simulink model "Motor_ctrl_INST"  (R2025b)
settings: Solver=ode15s  StartTime=0.0  StopTime=1  FixedStep=Ts/10  MaxStep=Tstep  RelTol=1e-3  AbsTol=1e-3  EnableMultiTasking=on
InitFcn:
  | if ~exist('flagwp')
  |     tic
  |     init_sim
  | end
  | mex Motor_ctrl.c User_functions/Src/*.c
StopFcn:
  | if ~exist('flagwp')
  |   elapsed_time=toc
  | end
values from neighbouring files (symbols this model uses):
  accel = 5000    [init_sim.m]
  Bm = 0    [init_sim.m]
  Clarke_inv = [1 0;-0.5 sqrt(3)/2;-0.5 -sqrt(3)/2]    [init_sim.m]
  Ctrl_strategy = 1    [init_sim.m]
  Ctrl_type = 3    [init_sim.m]
  dem = 1    [init_sim.m]
  dT = motorModel.SyreDrive.Converter.dT * 1e-6    [init_sim.m]
  expC = motorModel.IronPMLossMap_dq.expC    [init_sim.m]
  expH = motorModel.IronPMLossMap_dq.expH    [init_sim.m]
  expPM = motorModel.IronPMLossMap_dq.expPM    [init_sim.m]
  Fd0 = interp2(motorModel.FluxMap_dq.Id,motorModel.FluxMap_dq.Iq,motorModel.FluxMap_dq.Fd,0,0)    [init_sim.m]
  Fm = interp2(Idd,Iqq,Fdd,0,0)    [init_sim.m]
  HS_ctrl = 1    [init_sim.m]
  Id_dqt = interpn(motorModel.FluxMapInv_dqt.dataF.Fd,motorModel.FluxMapInv_dqt.dataF.Fq,motorModel.FluxMapInv_dqt.dataF.th,motorModel.FluxMapInv_dqt.dataF.Id,Fd_dqt,Fq_dqt,th_dqt,'cubic')    [init_sim.m]
  Id_fe = motorModel.IronPMLossMap_dq.Id    [init_sim.m]
  InitIntg_d = Fm*cos(th0)    [init_sim.m]
  InitIntg_q = Fm*sin(th0)    [init_sim.m]
  inj_waveform = 1    [init_sim.m]
  Iq_dqt = interpn(motorModel.FluxMapInv_dqt.dataF.Fd,motorModel.FluxMapInv_dqt.dataF.Fq,motorModel.FluxMapInv_dqt.dataF.th,motorModel.FluxMapInv_dqt.dataF.Iq,Fd_dqt,Fq_dqt,th_dqt,'cubic')    [init_sim.m]
  Iq_fe = motorModel.IronPMLossMap_dq.Iq    [init_sim.m]
  IronLoss = 1    [init_sim.m]
  J = motorModel.data.J    [init_sim.m]
  n0 = motorModel.IronPMLossMap_dq.n0    [init_sim.m]
  p = motorModel.data.p    [init_sim.m]
  Pfe_c = motorModel.IronPMLossMap_dq.Pfes_c + motorModel.IronPMLossMap_dq.Pfer_c    [init_sim.m]
  Pfe_h = motorModel.IronPMLossMap_dq.Pfes_h + motorModel.IronPMLossMap_dq.Pfer_h    [init_sim.m]
  Ppm = motorModel.IronPMLossMap_dq.Ppm    [init_sim.m]
  Quad_Maps = 2    [init_sim.m]
  SS_on = 1    [init_sim.m]
  T_dqt = interpn(motorModel.FluxMapInv_dqt.dataF.Fd,motorModel.FluxMapInv_dqt.dataF.Fq,motorModel.FluxMapInv_dqt.dataF.th,motorModel.FluxMapInv_dqt.dataF.T,Fd_dqt,Fq_dqt,th_dqt,'cubic')    [init_sim.m]
  Tf = 0    [init_sim.m]
  th0 = 0    [init_sim.m]
  th_max = max(motorModel.FluxMapInv_dqt.dataF.th,[],'all')    [init_sim.m]
  th_min = min(motorModel.FluxMapInv_dqt.dataF.th,[],'all')    [init_sim.m]
  Ts = 1/motorModel.SyreDrive.Converter.fPWM    [init_sim.m]
  Tv = 0    [init_sim.m]
  VDC = motorModel.data.Vdc    [init_sim.m]
undefined symbols (not defined in the file or in its folder): ACloss, eMotor, fD_pu_norm, fD_vct_max, fD_vct_ref, fQ_pu_norm, fQ_vct_max, fQ_vct_ref, iD_pu_norm, idRef, interpn, iQ_pu_norm, iqRef, J_rot, magnitude, motorModelType, nRef, sigbuilder_block, T0
libraries: nesl_utility x43, fl_lib x41, ee_lib x8, simulink x8, eeTransforms x1
(part 3 of 4)

== system Motor_ctrl_INST/Power block - Inverter + Motor/Circuital/Motor model/CCG model/Motor Model/Rs2/no AC loss ==
  Rs : Inport
  Current Sensor : fl_lib/Electrical/Electrical Sensors/Current Sensor
  PS-Simulink Converter : nesl_utility/PS-Simulink Converter  PhysicalDomain=network_engine_domain  SubClassName=ps_output  LeftPortType=input  RightPortType=output  PseudoPeriodic=off  Frequencies=[]  VectorFormat=inherit  Unit=inherit  AffineConversion=off
  PS-Simulink Converter1 : nesl_utility/PS-Simulink Converter  PhysicalDomain=network_engine_domain  SubClassName=ps_output  LeftPortType=input  RightPortType=output  PseudoPeriodic=off  Frequencies=[]  VectorFormat=inherit  Unit=inherit  AffineConversion=off
  Product : Product
  Resistor : fl_lib/Electrical/Electrical Elements/Resistor  R=ACloss.Rac(1) Ohm  i_specify=off  i_priority=None  i=0 A  i_nominal_specify=off  i_nominal_value=1  i_nominal_unit=A  v_specify=off  v_priority=None  v=0 V  v_nominal_specify=off  v_nominal_value=1  v_nominal_unit=V
  Terminator : Terminator
  Voltage Sensor : fl_lib/Electrical/Electrical Sensors/Voltage Sensor
  In : PMIOPort  Side=Left
  Out : PMIOPort  Port=2  Side=Right
  Pjs : Outport
  wires:
  PS-Simulink Converter/1 -> Product/1
  PS-Simulink Converter1/1 -> Product/2
  Product/1 -> Pjs/1
  Rs/1 -> Terminator/1
  connections:
  Resistor/LConn1 -- In/RConn1 -- Voltage Sensor/LConn1
  Current Sensor/RConn2 -- Out/RConn1
  Resistor/RConn1 -- Current Sensor/LConn1 -- Voltage Sensor/RConn2
  PS-Simulink Converter/LConn1 -- Voltage Sensor/RConn1
  PS-Simulink Converter1/LConn1 -- Current Sensor/RConn1

== system Motor_ctrl_INST/Power block - Inverter + Motor/Circuital/Motor model/CCG model/Motor Model/Rs2/yes AC loss ==
  Rs : Inport
  Current Sensor : fl_lib/Electrical/Electrical Sensors/Current Sensor
  PS-Simulink Converter : nesl_utility/PS-Simulink Converter  PhysicalDomain=network_engine_domain  SubClassName=ps_output  LeftPortType=input  RightPortType=output  PseudoPeriodic=off  Frequencies=[]  VectorFormat=inherit  Unit=inherit  AffineConversion=off
  PS-Simulink Converter1 : nesl_utility/PS-Simulink Converter  PhysicalDomain=network_engine_domain  SubClassName=ps_output  LeftPortType=input  RightPortType=output  PseudoPeriodic=off  Frequencies=[]  VectorFormat=inherit  Unit=inherit  AffineConversion=off
  Product : Product
  Simulink-PS Converter : nesl_utility/Simulink-PS Converter  PhysicalDomain=network_engine_domain  SubClassName=ps_input  LeftPortType=input  RightPortType=output  PseudoPeriodic=off  Frequencies=[]  NoiseDistribution=none  NoiseParameters=[]  Unit=1  AffineConversion=off  FilteringAndDerivatives=provide  SimscapeFilterOrder=1  InputFilterTimeConstant=0.001  UdotUserProvided=0
  Variable Resistor : fl_lib/Electrical/Electrical Elements/Variable Resistor  Rmin=0 Ohm  thermalEnable=false  thermal_mass=1 J/K  i_specify=off  i_priority=None  i=0 A  i_nominal_specify=off  i_nominal_value=1  i_nominal_unit=A  v_specify=off  v_priority=None  v=0 V  v_nominal_specify=off  v_nominal_value=1  v_nominal_unit=V  T_specify=off  T_priority=None  T=300 K  T_nominal_specify=off  T_nominal_value=1  T_nominal_unit=K
  Voltage Sensor : fl_lib/Electrical/Electrical Sensors/Voltage Sensor
  In : PMIOPort  Side=Left
  Out : PMIOPort  Port=2  Side=Right
  Pjs : Outport
  wires:
  PS-Simulink Converter1/1 -> Product/2
  PS-Simulink Converter/1 -> Product/1
  Product/1 -> Pjs/1
  Rs/1 -> Simulink-PS Converter/1
  connections:
  Variable Resistor/RConn1 -- Current Sensor/LConn1 -- Voltage Sensor/RConn2
  In/RConn1 -- Voltage Sensor/LConn1 -- Variable Resistor/LConn2
  Current Sensor/RConn2 -- Out/RConn1
  PS-Simulink Converter1/LConn1 -- Current Sensor/RConn1
  PS-Simulink Converter/LConn1 -- Voltage Sensor/RConn1
  Variable Resistor/LConn1 -- Simulink-PS Converter/RConn1

== system Motor_ctrl_INST/Power block - Inverter + Motor/Noncircuital/FM/Motor Model/Inverse Flux Maps/2D LUT/dq Model ==
  note: 1) Add Subsystem or Model blocks as valid variant choices.
      | 2) You cannot connect blocks at this level. At simulation, connectivity is automatically
      | determined, based on the active variant and port name matching.
  Vabc : Inport
  theta_elt : Inport  Port=2
  we : Inport  Port=3
  IPM : Subsystem  VariantControl=Quad_Maps==2
  PM-SyR : Subsystem  VariantControl=Quad_Maps==1
  SyR : Subsystem  VariantControl=Quad_Maps==0
  idq : Outport
  T : Outport  Port=2
  i0 : Outport  Port=3
  Fdq : Outport  Port=4

== system Motor_ctrl_INST/Power block - Inverter + Motor/Noncircuital/FM/Motor Model/Inverse Flux Maps/3D LUTs/Variant Subsystem ==
  note: 1) Add Subsystem or Model blocks as valid variant choices.
      | 2) You cannot connect blocks at this level. At simulation, connectivity is automatically
      | determined, based on the active variant and port name matching.
  Vabc : Inport
  theta_elt : Inport  Port=2
  we : Inport  Port=3
  IPM : Subsystem  VariantControl=Quad_Maps==2
  PM-SyR : Subsystem  VariantControl=Quad_Maps==1
  SyR : Subsystem  VariantControl=Quad_Maps==0
  idq : Outport
  T : Outport  Port=2
  i0 : Outport  Port=3
  Fdq : Outport  Port=4

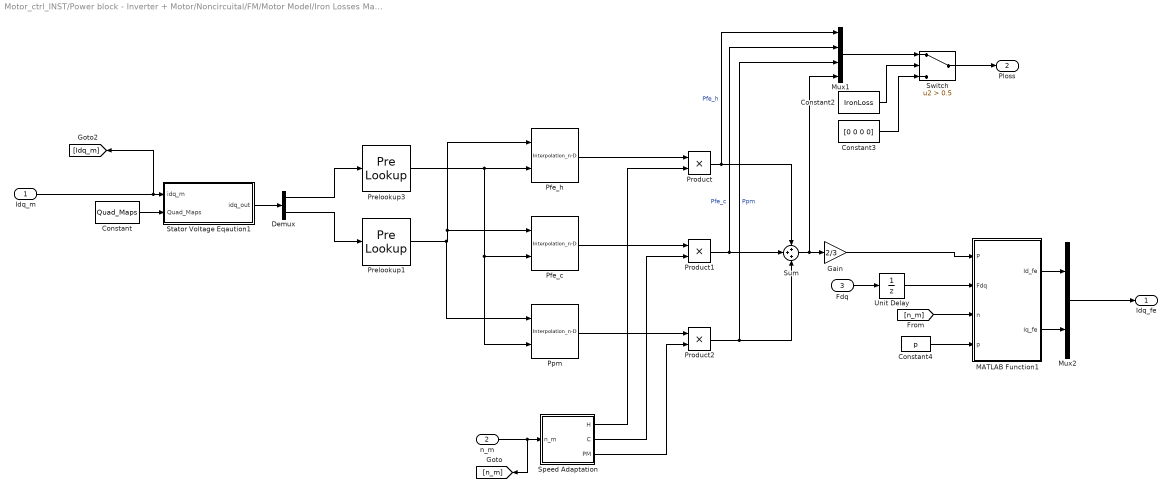
== system Motor_ctrl_INST/Power block - Inverter + Motor/Noncircuital/FM/Motor Model/Iron Losses Maps/Iron Losses/Iron loss Maps ==
  Idq_m : Inport
  n_m : Inport  Port=2
  Fdq : Inport  Port=3
  Constant : Constant  Value=Quad_Maps
  Constant2 : Constant  Value=IronLoss
  Constant3 : Constant  Value=[0 0 0 0]
  Constant4 : Constant  Value=p
  Demux : Demux  Outputs=2
  Gain : Gain  Gain=2/3
  MATLAB Function1 : MATLAB Function  TreatAsAtomicUnit=on
  Mux1 : Mux
  Mux2 : Mux  Inputs=2
  Pfe_c : Interpolation_n-D  Table=Pfe_c  RequireIndexFractionAsBus=on  InternalRulePriority=Speed
      settings: InputPortMap=u0,u1
  Pfe_h : Interpolation_n-D  Table=Pfe_h  RequireIndexFractionAsBus=on  InternalRulePriority=Speed
      settings: InputPortMap=u0,u1
  Ppm : Interpolation_n-D  Table=Ppm  RequireIndexFractionAsBus=on  InternalRulePriority=Speed
      settings: InputPortMap=u0,u1
  Prelookup1 : PreLookup  BreakpointsData=Iq_fe(:,1)  OutputSelection=Index and fraction as bus  ExtrapMethod=Linear
  Prelookup3 : PreLookup  BreakpointsData=Id_fe(1,:)  OutputSelection=Index and fraction as bus  ExtrapMethod=Linear
  Product : Product
  Product1 : Product
  Product2 : Product
  Speed Adaptation : Subsystem
  Stator Voltage Eqaution1 : MATLAB Function  TreatAsAtomicUnit=on
  Sum : Sum  Inputs=+++
  Switch : Switch  Criteria=u2 > Threshold  Threshold=0.5  SaturateOnIntegerOverflow=off  InputSameDT=off
  Unit Delay : UnitDelay  SampleTime=-1  HasFrameUpgradeWarning=on
  Idq_fe : Outport
  Ploss : Outport  Port=2
  wires:
  Product1/1 -> Mux1/2, Sum/2  "Pfe_c"
  Product2/1 -> Mux1/3, Sum/3  "Ppm"
  Pfe_h/1 -> Product/1
  Prelookup3/1 -> Ppm/2, Pfe_c/2, Pfe_h/2
  Speed Adaptation/1(H) -> Product/2
  n_m/1 -> Speed Adaptation/1(n_m), [n_m]
  Demux/1 -> Prelookup3/1
  Sum/1 -> Mux1/4, Gain/1
  Product/1 -> Sum/1, Mux1/1  "Pfe_h"
  Speed Adaptation/2(C) -> Product1/2
  Prelookup1/1 -> Ppm/1, Pfe_h/1, Pfe_c/1
  Pfe_c/1 -> Product1/1
  Ppm/1 -> Product2/1
  Demux/2 -> Prelookup1/1
  Speed Adaptation/3(PM) -> Product2/2
  Constant/1 -> Stator Voltage Eqaution1/2(Quad_Maps)
  Stator Voltage Eqaution1/1(idq_out) -> Demux/1
  Idq_m/1 -> [Idq_m], Stator Voltage Eqaution1/1(idq_m)
  Gain/1 -> MATLAB Function1/1(P)
  Fdq/1 -> Unit Delay/1
  [n_m] -> MATLAB Function1/3(n)
  Constant4/1 -> MATLAB Function1/4(p)
  MATLAB Function1/1(Id_fe) -> Mux2/1
  Mux2/1 -> Idq_fe/1
  Unit Delay/1 -> MATLAB Function1/2(Fdq)
  MATLAB Function1/2(Iq_fe) -> Mux2/2
  Mux1/1 -> Switch/1
  Constant2/1 -> Switch/2
  Switch/1 -> Ploss/1
  Constant3/1 -> Switch/3

== system Motor_ctrl_INST/Power block - Inverter + Motor/Circuital/Motor model/CCG model/Motor Model/Inverse Flux Maps/2D LUT/dq Model ==
  note: 1) Add Subsystem or Model blocks as valid variant choices.
      | 2) You cannot connect blocks at this level. At simulation, connectivity is automatically
      | determined, based on the active variant and port name matching.
  Fdq : Inport
  IPM : Subsystem  VariantControl=Quad_Maps==2
  PM-SyR : Subsystem  VariantControl=Quad_Maps==1
  SyR : Subsystem  VariantControl=Quad_Maps==0
  idq : Outport
  T : Outport  Port=2

== system Motor_ctrl_INST/Power block - Inverter + Motor/Circuital/Motor model/CCG model/Motor Model/Inverse Flux Maps/3D LUTs/Variant Subsystem ==
  note: 1) Add Subsystem or Model blocks as valid variant choices.
      | 2) You cannot connect blocks at this level. At simulation, connectivity is automatically
      | determined, based on the active variant and port name matching.
  Fdq : Inport
  theta_elt : Inport  Port=2
  IPM : Subsystem  VariantControl=Quad_Maps==2
  PM-SyR : Subsystem  VariantControl=Quad_Maps==1
  SyR : Subsystem  VariantControl=Quad_Maps==0
  idq : Outport
  T : Outport  Port=2

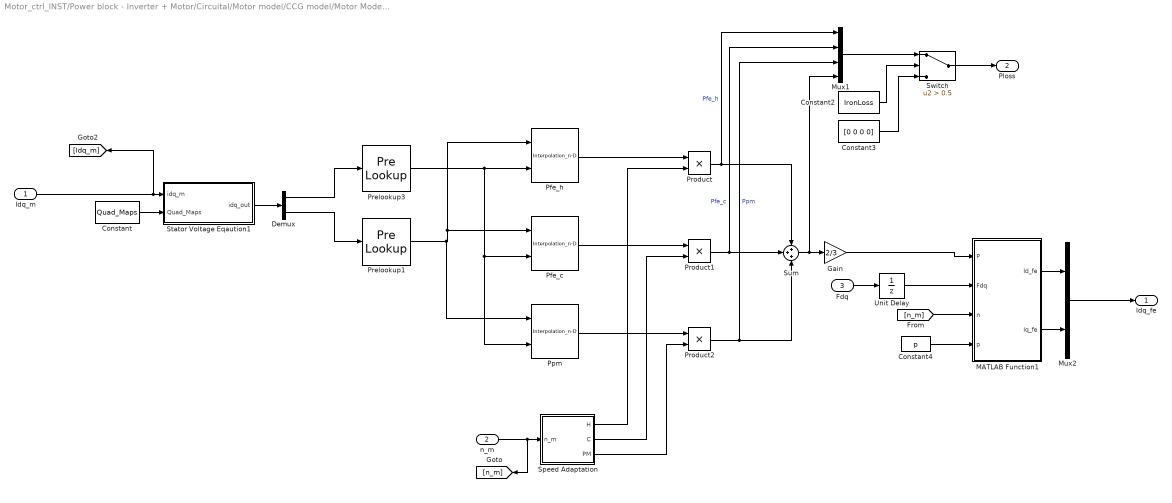
== system Motor_ctrl_INST/Power block - Inverter + Motor/Circuital/Motor model/CCG model/Motor Model/Iron Losses Maps/Iron Losses/Iron loss Maps ==
  Idq_m : Inport
  n_m : Inport  Port=2
  Fdq : Inport  Port=3
  Constant : Constant  Value=Quad_Maps
  Constant2 : Constant  Value=IronLoss
  Constant3 : Constant  Value=[0 0 0 0]
  Constant4 : Constant  Value=p
  Demux : Demux  Outputs=2
  Gain : Gain  Gain=2/3
  MATLAB Function1 : MATLAB Function  TreatAsAtomicUnit=on
  Mux1 : Mux
  Mux2 : Mux  Inputs=2
  Pfe_c : Interpolation_n-D  Table=Pfe_c  RequireIndexFractionAsBus=on  InternalRulePriority=Speed
      settings: InputPortMap=u0,u1
  Pfe_h : Interpolation_n-D  Table=Pfe_h  RequireIndexFractionAsBus=on  InternalRulePriority=Speed
      settings: InputPortMap=u0,u1
  Ppm : Interpolation_n-D  Table=Ppm  RequireIndexFractionAsBus=on  InternalRulePriority=Speed
      settings: InputPortMap=u0,u1
  Prelookup1 : PreLookup  BreakpointsData=Iq_fe(:,1)  OutputSelection=Index and fraction as bus  ExtrapMethod=Linear
  Prelookup3 : PreLookup  BreakpointsData=Id_fe(1,:)  OutputSelection=Index and fraction as bus  ExtrapMethod=Linear
  Product : Product
  Product1 : Product
  Product2 : Product
  Speed Adaptation : Subsystem
  Stator Voltage Eqaution1 : MATLAB Function  TreatAsAtomicUnit=on
  Sum : Sum  Inputs=+++
  Switch : Switch  Criteria=u2 > Threshold  Threshold=0.5  SaturateOnIntegerOverflow=off  InputSameDT=off
  Unit Delay : UnitDelay  SampleTime=-1  HasFrameUpgradeWarning=on
  Idq_fe : Outport
  Ploss : Outport  Port=2
  wires:
  Product1/1 -> Mux1/2, Sum/2  "Pfe_c"
  Product2/1 -> Mux1/3, Sum/3  "Ppm"
  Pfe_h/1 -> Product/1
  Prelookup3/1 -> Ppm/2, Pfe_c/2, Pfe_h/2
  Speed Adaptation/1(H) -> Product/2
  n_m/1 -> Speed Adaptation/1(n_m), [n_m]
  Demux/1 -> Prelookup3/1
  Sum/1 -> Mux1/4, Gain/1
  Product/1 -> Sum/1, Mux1/1  "Pfe_h"
  Speed Adaptation/2(C) -> Product1/2
  Prelookup1/1 -> Ppm/1, Pfe_h/1, Pfe_c/1
  Pfe_c/1 -> Product1/1
  Ppm/1 -> Product2/1
  Demux/2 -> Prelookup1/1
  Speed Adaptation/3(PM) -> Product2/2
  Constant/1 -> Stator Voltage Eqaution1/2(Quad_Maps)
  Stator Voltage Eqaution1/1(idq_out) -> Demux/1
  Idq_m/1 -> [Idq_m], Stator Voltage Eqaution1/1(idq_m)
  Gain/1 -> MATLAB Function1/1(P)
  Fdq/1 -> Unit Delay/1
  [n_m] -> MATLAB Function1/3(n)
  Constant4/1 -> MATLAB Function1/4(p)
  MATLAB Function1/1(Id_fe) -> Mux2/1
  Mux2/1 -> Idq_fe/1
  Unit Delay/1 -> MATLAB Function1/2(Fdq)
  MATLAB Function1/2(Iq_fe) -> Mux2/2
  Mux1/1 -> Switch/1
  Constant2/1 -> Switch/2
  Switch/1 -> Ploss/1
  Constant3/1 -> Switch/3

== system Motor_ctrl_INST/Power block - Inverter + Motor/Noncircuital/FM/Motor Model/Inverse Flux Maps/2D LUT/dq Model/IPM ==
  Vabc : Inport
  theta_elt : Inport  Port=2
  we : Inport  Port=3
  Add : Sum  Inputs=-+-
  Constant : Constant  Value=0
  Demux1 : Demux  Outputs=3
  "Fdq -> idq" : Subsystem
  Gain1 : Gain  Gain=J_rot  Multiplication=Matrix(K*u)
  Gain3 : Gain  Gain=1/p
  Integrator : Integrator  InitialCondition=[Fd0 0]
  Mux1 : Mux  Inputs=2
  Product : Product
  Product2 : Product
  Subsystem1 : Subsystem
  Terminator : Terminator
  ab->dq1 : Subsystem
      mask Display: disp('A(-theta)')
  abc->ab0 : Subsystem
  idq : Outport
  T : Outport  Port=2
  i0 : Outport  Port=3
  Fdq : Outport  Port=4
  wires:
  Add/1 -> Integrator/1
  Demux1/2 -> Mux1/2
  we/1 -> Product/2
  [Rs] -> Product2/1
  Product2/1 -> Add/1
  "Fdq -> idq"/2(T) -> T/1
  Demux1/1 -> Mux1/1
  abc->ab0/1(eab0) -> Demux1/1
  "Fdq -> idq"/1(idq) -> Product2/2, idq/1
  Product/1 -> Add/3
  theta_elt/1 -> Gain3/1
  ab->dq1/1(X_dq) -> Add/2
  Vabc/1 -> abc->ab0/1(eabc)
  Integrator/1 -> "Fdq -> idq"/1(Fdq), Fdq/1, Gain1/1
  Gain3/1 -> Subsystem1/1(theta_r)
  Mux1/1 -> ab->dq1/1(X_ab)
  Gain1/1 -> Product/1
  Subsystem1/1(SinCos) -> ab->dq1/2(sin,cos)
  Constant/1 -> i0/1
  Demux1/3 -> Terminator/1

== system Motor_ctrl_INST/Power block - Inverter + Motor/Noncircuital/FM/Motor Model/Inverse Flux Maps/2D LUT/dq Model/PM-SyR ==
  Vabc : Inport
  theta_elt : Inport  Port=2
  we : Inport  Port=3
  Add : Sum  Inputs=-+-
  Constant : Constant  Value=0
  Demux1 : Demux  Outputs=3
  "Fdq -> idq" : Subsystem
  Gain1 : Gain  Gain=J_rot  Multiplication=Matrix(K*u)
  Gain3 : Gain  Gain=1/p
  Integrator : Integrator  InitialCondition=[Fd0 0]
  Mux1 : Mux  Inputs=2
  Product : Product
  Product2 : Product
  Subsystem1 : Subsystem
  Terminator : Terminator
  ab->dq1 : Subsystem
      mask Display: disp('A(-theta)')
  abc->ab0 : Subsystem
  idq : Outport
  T : Outport  Port=2
  i0 : Outport  Port=3
  Fdq : Outport  Port=4
  wires:
  Subsystem1/1(SinCos) -> ab->dq1/2(sin,cos)
  Product/1 -> Add/3
  theta_elt/1 -> Gain3/1
  Mux1/1 -> ab->dq1/1(X_ab)
  Integrator/1 -> "Fdq -> idq"/1(Fdq), Fdq/1, Gain1/1
  Gain1/1 -> Product/1
  Vabc/1 -> abc->ab0/1(eabc)
  Gain3/1 -> Subsystem1/1(theta_r)
  ab->dq1/1(X_dq) -> Add/2
  abc->ab0/1(eab0) -> Demux1/1
  "Fdq -> idq"/1(idq) -> Product2/2, idq/1
  Demux1/1 -> Mux1/1
  Add/1 -> Integrator/1
  [Rs] -> Product2/1
  Demux1/2 -> Mux1/2
  Product2/1 -> Add/1
  we/1 -> Product/2
  "Fdq -> idq"/2(T) -> T/1
  Constant/1 -> i0/1
  Demux1/3 -> Terminator/1

== system Motor_ctrl_INST/Power block - Inverter + Motor/Noncircuital/FM/Motor Model/Inverse Flux Maps/2D LUT/dq Model/SyR ==
  Vabc : Inport
  theta_elt : Inport  Port=2
  we : Inport  Port=3
  Add : Sum  Inputs=-+-
  Constant : Constant  Value=0
  Demux1 : Demux  Outputs=3
  "Fdq -> idq" : Subsystem
  Gain1 : Gain  Gain=J_rot  Multiplication=Matrix(K*u)
  Gain3 : Gain  Gain=1/p
  Integrator : Integrator  InitialCondition=[Fd0 0]
  Mux1 : Mux  Inputs=2
  Product : Product
  Product2 : Product
  Subsystem1 : Subsystem
  Terminator : Terminator
  ab->dq1 : Subsystem
      mask Display: disp('A(-theta)')
  abc->ab0 : Subsystem
  idq : Outport
  T : Outport  Port=2
  i0 : Outport  Port=3
  Fdq : Outport  Port=4
  wires:
  Subsystem1/1(SinCos) -> ab->dq1/2(sin,cos)
  Product/1 -> Add/3
  theta_elt/1 -> Gain3/1
  Mux1/1 -> ab->dq1/1(X_ab)
  Integrator/1 -> "Fdq -> idq"/1(Fdq), Fdq/1, Gain1/1
  Gain1/1 -> Product/1
  Vabc/1 -> abc->ab0/1(eabc)
  Gain3/1 -> Subsystem1/1(theta_r)
  ab->dq1/1(X_dq) -> Add/2
  abc->ab0/1(eab0) -> Demux1/1
  "Fdq -> idq"/1(idq) -> Product2/2, idq/1
  Demux1/1 -> Mux1/1
  Add/1 -> Integrator/1
  [Rs] -> Product2/1
  Demux1/2 -> Mux1/2
  "Fdq -> idq"/2(T) -> T/1
  Product2/1 -> Add/1
  we/1 -> Product/2
  Constant/1 -> i0/1
  Demux1/3 -> Terminator/1

== system Motor_ctrl_INST/Power block - Inverter + Motor/Noncircuital/FM/Motor Model/Inverse Flux Maps/3D LUTs/Variant Subsystem/IPM ==
  Vabc : Inport
  theta_elt : Inport  Port=2
  we : Inport  Port=3
  Add : Sum  Inputs=-+-
  Constant : Constant  Value=0
  Demux1 : Demux  Outputs=3
  "Fdq -> idq" : Subsystem
      settings: PortSchema="{\"entries\":[{\"content\":{\"sides\":[{\"content\":{\"connectorIds\":[\"In1\"]},\"type\":\"ConnectorPlacement.EquallySpacedRectSide\",\"uuid\":\"c4c89702-6ed2-4f3f-ac47-63a7def21c28\"},{\"content\":{\"connectorIds\":[\"Out1\",\"Out2\"],\"side\":\"RIGHT\"},\"type\":\"ConnectorPlacement.EquallySpacedRectSide\",\"uuid\":\"78e6e96f-e01c-41b0-b9cc-2e557d2d3e77\"},{\"content\":{\"side\":\"TOP\"},\"type\":\"ConnectorPlacement.EquallySpacedRectSide\",\"uuid\":\"5ba1a012-9577-477d-841c-cd762f3f0080\"},{\"content\":{\"connectorIds\":[\"In2\"],\"side\":\"BOTTOM\"},\"type\":\"ConnectorPlacement.EquallySpacedRectSide\",\"uuid\":\"5a42fb6c-9e1a-4def-8312-83961c7d32ea\"}]},\"type\":\"ConnectorPlacement.EquallySpacedConnector\",\"uuid\":\"db03f8b0-b4f5-4aab-82fc-8dea803a4789\"}],\"packageUris\":[\"http://schema.mathworks.com/mf0/Connector/R2020b\"],\"version\":\"1.0\"}"
  Gain1 : Gain  Gain=J_rot  Multiplication=Matrix(K*u)
  Gain3 : Gain  Gain=1/p
  Integrator : Integrator  InitialCondition=[Fd0 0]
  Mux1 : Mux  Inputs=2
  Product : Product
  Product1 : Product
  Subsystem1 : Subsystem
  Terminator : Terminator
  ab->dq1 : Subsystem
      mask Display: disp('A(-theta)')
  abc->ab0 : Subsystem
  idq : Outport
  T : Outport  Port=2
  i0 : Outport  Port=3
  Fdq : Outport  Port=4
  wires:
  theta_elt/1 -> "Fdq -> idq"/2(th_e), Gain3/1
  Product1/1 -> Add/1
  Gain1/1 -> Product/1
  we/1 -> Product/2
  Product/1 -> Add/3
  Add/1 -> Integrator/1
  Integrator/1 -> Fdq/1, "Fdq -> idq"/1(Fdq), Gain1/1
  "Fdq -> idq"/1(idq) -> Product1/2, idq/1
  "Fdq -> idq"/2(T) -> T/1
  [Rs] -> Product1/1
  Vabc/1 -> abc->ab0/1(eabc)
  Gain3/1 -> Subsystem1/1(theta_r)
  abc->ab0/1(eab0) -> Demux1/1
  Subsystem1/1(SinCos) -> ab->dq1/2(sin,cos)
  Demux1/2 -> Mux1/2
  Mux1/1 -> ab->dq1/1(X_ab)
  Demux1/1 -> Mux1/1
  ab->dq1/1(X_dq) -> Add/2
  Constant/1 -> i0/1
  Demux1/3 -> Terminator/1

== system Motor_ctrl_INST/Power block - Inverter + Motor/Noncircuital/FM/Motor Model/Inverse Flux Maps/3D LUTs/Variant Subsystem/PM-SyR ==
  Vabc : Inport
  theta_elt : Inport  Port=2
  we : Inport  Port=3
  Add : Sum  Inputs=-+-
  Constant : Constant  Value=0
  Demux1 : Demux  Outputs=3
  "Fdq -> idq" : Subsystem
      settings: PortSchema="{\"entries\":[{\"content\":{\"sides\":[{\"content\":{\"connectorIds\":[\"In1\"]},\"type\":\"ConnectorPlacement.EquallySpacedRectSide\",\"uuid\":\"658e0025-c3b4-4188-99f2-cbeabc2b5232\"},{\"content\":{\"connectorIds\":[\"Out1\",\"Out2\"],\"side\":\"RIGHT\"},\"type\":\"ConnectorPlacement.EquallySpacedRectSide\",\"uuid\":\"553a685c-efe6-4f4b-af8f-d6d55fb3aed3\"},{\"content\":{\"side\":\"TOP\"},\"type\":\"ConnectorPlacement.EquallySpacedRectSide\",\"uuid\":\"e1cc6d12-3f22-4810-870a-14518fddf4c6\"},{\"content\":{\"connectorIds\":[\"In2\"],\"side\":\"BOTTOM\"},\"type\":\"ConnectorPlacement.EquallySpacedRectSide\",\"uuid\":\"8fa353db-c23e-4667-be44-c63eaefe25e8\"}]},\"type\":\"ConnectorPlacement.EquallySpacedConnector\",\"uuid\":\"5d87f386-f61d-410e-9580-edc792fe8ce3\"}],\"packageUris\":[\"http://schema.mathworks.com/mf0/Connector/R2020b\"],\"version\":\"1.0\"}"
  Gain1 : Gain  Gain=J_rot  Multiplication=Matrix(K*u)
  Gain3 : Gain  Gain=1/p
  Integrator : Integrator  InitialCondition=[Fd0 0]
  Mux1 : Mux  Inputs=2
  Product : Product
  Product1 : Product
  Subsystem1 : Subsystem
  Terminator : Terminator
  ab->dq1 : Subsystem
      mask Display: disp('A(-theta)')
  abc->ab0 : Subsystem
  idq : Outport
  T : Outport  Port=2
  i0 : Outport  Port=3
  Fdq : Outport  Port=4
  wires:
  we/1 -> Product/2
  Subsystem1/1(SinCos) -> ab->dq1/2(sin,cos)
  Mux1/1 -> ab->dq1/1(X_ab)
  Gain1/1 -> Product/1
  Product/1 -> Add/3
  abc->ab0/1(eab0) -> Demux1/1
  ab->dq1/1(X_dq) -> Add/2
  [Rs] -> Product1/1
  "Fdq -> idq"/2(T) -> T/1
  Demux1/1 -> Mux1/1
  Product1/1 -> Add/1
  Demux1/3 -> Terminator/1
  Gain3/1 -> Subsystem1/1(theta_r)
  Integrator/1 -> "Fdq -> idq"/1(Fdq), Fdq/1, Gain1/1
  "Fdq -> idq"/1(idq) -> Product1/2, idq/1
  Demux1/2 -> Mux1/2
  Add/1 -> Integrator/1
  Vabc/1 -> abc->ab0/1(eabc)
  theta_elt/1 -> Gain3/1, "Fdq -> idq"/2(theta_elt)
  Constant/1 -> i0/1

== system Motor_ctrl_INST/Power block - Inverter + Motor/Noncircuital/FM/Motor Model/Inverse Flux Maps/3D LUTs/Variant Subsystem/SyR ==
  Vabc : Inport
  theta_elt : Inport  Port=2
  we : Inport  Port=3
  Add : Sum  Inputs=-+-
  Constant : Constant  Value=0
  Demux1 : Demux  Outputs=3
  "Fdq -> idq" : Subsystem
      settings: PortSchema="{\"entries\":[{\"content\":{\"sides\":[{\"content\":{\"connectorIds\":[\"In1\"]},\"type\":\"ConnectorPlacement.EquallySpacedRectSide\",\"uuid\":\"658e0025-c3b4-4188-99f2-cbeabc2b5232\"},{\"content\":{\"connectorIds\":[\"Out1\",\"Out2\"],\"side\":\"RIGHT\"},\"type\":\"ConnectorPlacement.EquallySpacedRectSide\",\"uuid\":\"553a685c-efe6-4f4b-af8f-d6d55fb3aed3\"},{\"content\":{\"side\":\"TOP\"},\"type\":\"ConnectorPlacement.EquallySpacedRectSide\",\"uuid\":\"e1cc6d12-3f22-4810-870a-14518fddf4c6\"},{\"content\":{\"connectorIds\":[\"In2\"],\"side\":\"BOTTOM\"},\"type\":\"ConnectorPlacement.EquallySpacedRectSide\",\"uuid\":\"ed75ffcc-b3fe-4912-8b15-453be7565ae7\"}]},\"type\":\"ConnectorPlacement.EquallySpacedConnector\",\"uuid\":\"5d87f386-f61d-410e-9580-edc792fe8ce3\"}],\"packageUris\":[\"http://schema.mathworks.com/mf0/Connector/R2020b\"],\"version\":\"1.0\"}"
  Gain1 : Gain  Gain=J_rot  Multiplication=Matrix(K*u)
  Gain3 : Gain  Gain=1/p
  Integrator : Integrator  InitialCondition=[Fd0 0]
  Mux1 : Mux  Inputs=2
  Product : Product
  Product1 : Product
  Subsystem1 : Subsystem
  Terminator : Terminator
  ab->dq1 : Subsystem
      mask Display: disp('A(-theta)')
  abc->ab0 : Subsystem
  idq : Outport
  T : Outport  Port=2
  i0 : Outport  Port=3
  Fdq : Outport  Port=4
  wires:
  we/1 -> Product/2
  Subsystem1/1(SinCos) -> ab->dq1/2(sin,cos)
  Mux1/1 -> ab->dq1/1(X_ab)
  Gain1/1 -> Product/1
  Product/1 -> Add/3
  abc->ab0/1(eab0) -> Demux1/1
  ab->dq1/1(X_dq) -> Add/2
  [Rs] -> Product1/1
  "Fdq -> idq"/2(T) -> T/1
  Demux1/1 -> Mux1/1
  Product1/1 -> Add/1
  Gain3/1 -> Subsystem1/1(theta_r)
  Integrator/1 -> "Fdq -> idq"/1(Fdq), Fdq/1, Gain1/1
  "Fdq -> idq"/1(idq) -> Product1/2, idq/1
  Demux1/2 -> Mux1/2
  Add/1 -> Integrator/1
  Vabc/1 -> abc->ab0/1(eabc)
  theta_elt/1 -> "Fdq -> idq"/2(theta_elt), Gain3/1
  Constant/1 -> i0/1
  Demux1/3 -> Terminator/1

== system Motor_ctrl_INST/Power block - Inverter + Motor/Noncircuital/FM/Motor Model/Iron Losses Maps/Iron Losses/Iron loss Maps/Speed Adaptation ==
  n_m : Inport
  Constant : Constant  Value=n0
  Constant1 : Constant  Value=expC
  Constant2 : Constant  Value=expH
  Constant3 : Constant  Value=expPM
  Divide : Product  Inputs=*/
  Math Function : Math  Operator=pow  SignedPower=on
  Math Function1 : Math  Operator=pow  SignedPower=on
  Math Function2 : Math  Operator=pow  SignedPower=on
  H : Outport
  C : Outport  Port=2
  PM : Outport  Port=3
  wires:
  Math Function2/1 -> PM/1
  Math Function/1 -> H/1
  Constant1/1 -> Math Function1/2
  Divide/1 -> Math Function/1, Math Function1/1, Math Function2/1
  Math Function1/1 -> C/1
  Constant/1 -> Divide/2
  Constant2/1 -> Math Function/2
  Constant3/1 -> Math Function2/2
  n_m/1 -> Divide/1

== system Motor_ctrl_INST/Power block - Inverter + Motor/Circuital/Motor model/CCG model/Motor Model/Inverse Flux Maps/2D LUT/dq Model/IPM ==
  Fdq : Inport
  1-D Lookup Table : Lookup_n-D  NumberOfTableDimensions=1  BreakpointsForDimension1=fD_vct_ref  Table=fQ_vct_max  InternalRulePriority=Speed  RndMeth=Simplest
  Abs1 : Abs  SaturateOnIntegerOverflow=off
  Bias : Bias  Bias=-fD_vct_ref(1)  SaturateOnIntegerOverflow=off
  Constant : Constant  Value=fD_vct_ref(end)-fD_vct_ref(1)
  Demux : Demux  Outputs=2
  Divide : Product  Inputs=*/
  Divide1 : Product  Inputs=/*
  Id_pu : Lookup_n-D  BreakpointsForDimension1=fQ_pu_norm(:,1)  BreakpointsForDimension2=fD_pu_norm(1,:)  Table=iD_pu_norm  InternalRulePriority=Speed  RndMeth=Simplest
      settings: InputPortMap=u0,u1
  Iq_pu : Lookup_n-D  BreakpointsForDimension1=fQ_pu_norm(:,1)  BreakpointsForDimension2=fD_pu_norm(1,:)  Table=iQ_pu_norm  InternalRulePriority=Speed  RndMeth=Simplest
      settings: InputPortMap=u0,u1
  Mux : Mux  Inputs=2
  Product1 : Product
  Saturation : Saturate  UpperLimit=fD_vct_ref(end)  LowerLimit=fD_vct_ref(1)
  Saturation Dynamic : simulink/Discontinuities/Saturation Dynamic  OutMin=[]  OutMax=[]  OutDataTypeStr=Inherit: Same as second input  OutDataType=fixdt(1, 16)  OutScaling=2^-10  DoSatur=off
  Sign1 : Signum
  Torque calculation : Subsystem
  idq : Outport
  T : Outport  Port=2
  wires:
  Iq_pu/1 -> Product1/1
  Demux/2 -> Sign1/1, Abs1/1
  Sign1/1 -> Product1/2
  Fdq/1 -> Torque calculation/2(Fdq), Demux/1
  Mux/1 -> Torque calculation/1(Idq), idq/1
  Bias/1 -> Divide/1
  Product1/1 -> Mux/2  "iq_pu"
  Constant/1 -> Divide/2
  1-D Lookup Table/1 -> Divide1/1, Saturation Dynamic/1
  Torque calculation/1(Tm) -> T/1
  Saturation Dynamic/1 -> Divide1/2
  Abs1/1 -> Saturation Dynamic/3, Saturation Dynamic/2
  Divide1/1 -> Id_pu/1, Iq_pu/1
  Demux/1 -> Saturation/1
  Divide/1 -> Iq_pu/2, Id_pu/2
  Saturation/1 -> Bias/1, 1-D Lookup Table/1
  Id_pu/1 -> Mux/1  "iq_pu"

== system Motor_ctrl_INST/Power block - Inverter + Motor/Circuital/Motor model/CCG model/Motor Model/Inverse Flux Maps/2D LUT/dq Model/PM-SyR ==
  Fdq : Inport
  1-D Lookup Table : Lookup_n-D  NumberOfTableDimensions=1  BreakpointsForDimension1=fQ_vct_ref  Table=fD_vct_max  InternalRulePriority=Speed  RndMeth=Simplest
  Abs : Abs  SaturateOnIntegerOverflow=off
  Bias : Bias  Bias=-fQ_vct_ref(1)  SaturateOnIntegerOverflow=off
  Constant : Constant  Value=fQ_vct_ref(end)-fQ_vct_ref(1)
  Demux : Demux  Outputs=2
  Divide : Product  Inputs=*/
  Divide1 : Product  Inputs=/*
  Id_pu : Lookup_n-D  BreakpointsForDimension1=fQ_pu_norm(:,1)  BreakpointsForDimension2=fD_pu_norm(1,:)  Table=iD_pu_norm  InternalRulePriority=Speed  RndMeth=Simplest
      settings: InputPortMap=u0,u1
  Iq_pu : Lookup_n-D  BreakpointsForDimension1=fQ_pu_norm(:,1)  BreakpointsForDimension2=fD_pu_norm(1,:)  Table=iQ_pu_norm  InternalRulePriority=Speed  RndMeth=Simplest
      settings: InputPortMap=u0,u1
  Mux : Mux  Inputs=2
  Product2 : Product
  Saturation : Saturate  UpperLimit=fQ_vct_ref(end)  LowerLimit=fQ_vct_ref(1)
  Saturation Dynamic : simulink/Discontinuities/Saturation Dynamic  OutMin=[]  OutMax=[]  OutDataTypeStr=Inherit: Same as second input  OutDataType=fixdt(1, 16)  OutScaling=2^-10  DoSatur=off
  Sign2 : Signum
  Torque calculation : Subsystem
  idq : Outport
  T : Outport  Port=2
  wires:
  Torque calculation/1(Tm) -> T/1
  Saturation/1 -> Bias/1, 1-D Lookup Table/1
  Bias/1 -> Divide/1
  Saturation Dynamic/1 -> Divide1/2
  Iq_pu/1 -> Mux/2  "iq_pu"
  1-D Lookup Table/1 -> Divide1/1, Saturation Dynamic/1
  Sign2/1 -> Product2/1
  Fdq/1 -> Torque calculation/2(Fdq), Demux/1
  Id_pu/1 -> Product2/2
  Product2/1 -> Mux/1  "id_pu"
  Mux/1 -> idq/1, Torque calculation/1(Idq)
  Constant/1 -> Divide/2
  Abs/1 -> Saturation Dynamic/3, Saturation Dynamic/2
  Demux/2 -> Saturation/1
  Demux/1 -> Sign2/1, Abs/1
  Divide1/1 -> Id_pu/2, Iq_pu/2
  Divide/1 -> Iq_pu/1, Id_pu/1

== system Motor_ctrl_INST/Power block - Inverter + Motor/Circuital/Motor model/CCG model/Motor Model/Inverse Flux Maps/2D LUT/dq Model/SyR ==
  Fdq : Inport
  1-D Lookup Table : Lookup_n-D  NumberOfTableDimensions=1  BreakpointsForDimension1=fD_vct_ref  Table=fQ_vct_max  InternalRulePriority=Speed  RndMeth=Simplest
  Abs1 : Abs  SaturateOnIntegerOverflow=off
  Abs2 : Abs  SaturateOnIntegerOverflow=off
  Bias : Bias  Bias=-fD_vct_ref(1)  SaturateOnIntegerOverflow=off
  Constant : Constant  Value=fD_vct_ref(end)-fD_vct_ref(1)
  Demux : Demux  Outputs=2
  Divide : Product  Inputs=*/
  Divide1 : Product  Inputs=/*
  Id_pu : Lookup_n-D  BreakpointsForDimension1=fQ_pu_norm(:,1)  BreakpointsForDimension2=fD_pu_norm(1,:)  Table=iD_pu_norm  InternalRulePriority=Speed  RndMeth=Simplest
      settings: InputPortMap=u0,u1
  Iq_pu : Lookup_n-D  BreakpointsForDimension1=fQ_pu_norm(:,1)  BreakpointsForDimension2=fD_pu_norm(1,:)  Table=iQ_pu_norm  InternalRulePriority=Speed  RndMeth=Simplest
      settings: InputPortMap=u0,u1
  Mux : Mux  Inputs=2
  Product1 : Product
  Product2 : Product
  Saturation : Saturate  UpperLimit=fD_vct_ref(end)  LowerLimit=fD_vct_ref(1)
  Saturation Dynamic : simulink/Discontinuities/Saturation Dynamic  OutMin=[]  OutMax=[]  OutDataTypeStr=Inherit: Same as second input  OutDataType=fixdt(1, 16)  OutScaling=2^-10  DoSatur=off
  Sign1 : Signum
  Sign2 : Signum
  Torque calculation : Subsystem
  idq : Outport
  T : Outport  Port=2
  wires:
  Fdq/1 -> Torque calculation/2(Fdq), Demux/1
  Mux/1 -> Torque calculation/1(Idq), idq/1
  Product1/1 -> Mux/2  "iq_pu"
  Constant/1 -> Divide/2
  Bias/1 -> Divide/1
  Divide/1 -> Iq_pu/2, Id_pu/2
  Demux/2 -> Sign1/1, Abs1/1
  Saturation/1 -> Bias/1, 1-D Lookup Table/1
  Divide1/1 -> Id_pu/1, Iq_pu/1
  Demux/1 -> Abs2/1, Sign2/1
  Abs1/1 -> Saturation Dynamic/3, Saturation Dynamic/2
  Sign1/1 -> Product1/2
  Iq_pu/1 -> Product1/1
  1-D Lookup Table/1 -> Divide1/1, Saturation Dynamic/1
  Saturation Dynamic/1 -> Divide1/2
  Id_pu/1 -> Product2/2
  Product2/1 -> Mux/1  "iq_pu"
  Abs2/1 -> Saturation/1
  Sign2/1 -> Product2/1
  Torque calculation/1(Tm) -> T/1

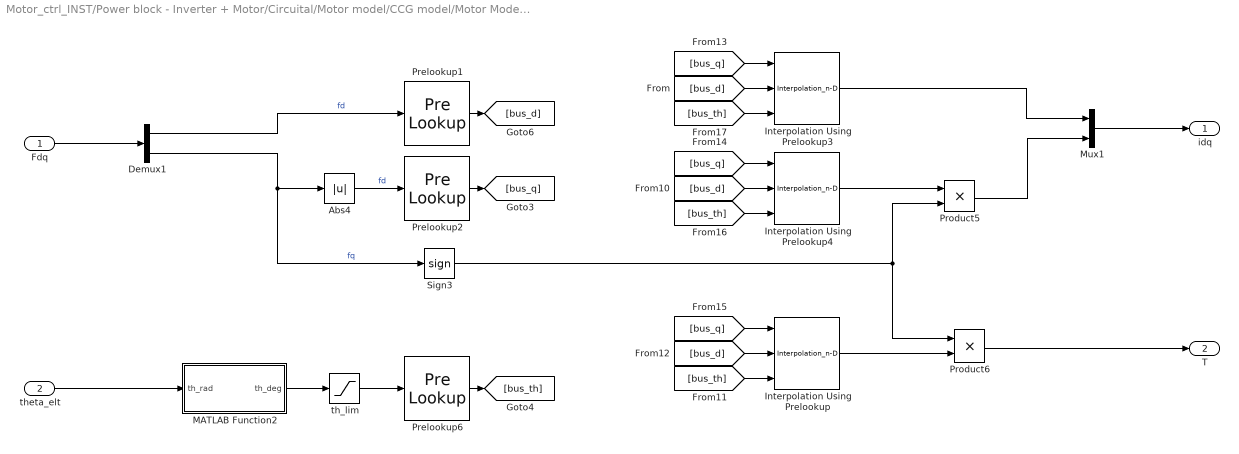
== system Motor_ctrl_INST/Power block - Inverter + Motor/Circuital/Motor model/CCG model/Motor Model/Inverse Flux Maps/3D LUTs/Variant Subsystem/IPM ==
  Fdq : Inport
  theta_elt : Inport  Port=2
  Abs4 : Abs  SaturateOnIntegerOverflow=off
  Demux1 : Demux  Outputs=2
  Interpolation Using Prelookup : Interpolation_n-D  NumberOfTableDimensions=3  Table=T_dqt  LookupTableObject=T_th  RequireIndexFractionAsBus=on  InternalRulePriority=Speed
      settings: InputPortMap=u0,u1,u2
  Interpolation Using Prelookup3 : Interpolation_n-D  NumberOfTableDimensions=3  Table=Id_dqt  RequireIndexFractionAsBus=on  InternalRulePriority=Speed
      settings: InputPortMap=u0,u1,u2
  Interpolation Using Prelookup4 : Interpolation_n-D  NumberOfTableDimensions=3  Table=Iq_dqt  RequireIndexFractionAsBus=on  InternalRulePriority=Speed
      settings: InputPortMap=u0,u1,u2
  MATLAB Function2 : MATLAB Function  TreatAsAtomicUnit=on
  Mux1 : Mux  Inputs=2
  Prelookup1 : PreLookup  BreakpointsData=Fd_v  OutputSelection=Index and fraction as bus  ExtrapMethod=Linear
  Prelookup2 : PreLookup  BreakpointsData=Fq_v  OutputSelection=Index and fraction as bus  ExtrapMethod=Linear
  Prelookup6 : PreLookup  BreakpointsData=th_v  OutputSelection=Index and fraction as bus  ExtrapMethod=Linear
  Product5 : Product
  Product6 : Product
  Sign3 : Signum
  th_lim : Saturate  UpperLimit=th_max  LowerLimit=th_min  ZeroCross=off
  idq : Outport
  T : Outport  Port=2
  wires:
  theta_elt/1 -> MATLAB Function2/1(th_rad)
  Sign3/1 -> Product6/1, Product5/2
  Interpolation Using Prelookup3/1 -> Mux1/1
  Product5/1 -> Mux1/2
  Product6/1 -> T/1
  Interpolation Using Prelookup4/1 -> Product5/1
  Abs4/1 -> Prelookup2/1  "fd"
  MATLAB Function2/1(th_deg) -> th_lim/1
  [bus_d] -> Interpolation Using Prelookup3/2
  [bus_d] -> Interpolation Using Prelookup4/2
  Prelookup1/1 -> [bus_d]
  [bus_q] -> Interpolation Using Prelookup/1
  Demux1/2 -> Sign3/1, Abs4/1  "fq"
  [bus_th] -> Interpolation Using Prelookup/3
  [bus_q] -> Interpolation Using Prelookup4/1
  [bus_d] -> Interpolation Using Prelookup/2
  [bus_q] -> Interpolation Using Prelookup3/1
  [bus_th] -> Interpolation Using Prelookup4/3
  Demux1/1 -> Prelookup1/1  "fd"
  th_lim/1 -> Prelookup6/1
  Prelookup6/1 -> [bus_th]
  [bus_th] -> Interpolation Using Prelookup3/3
  Prelookup2/1 -> [bus_q]
  Mux1/1 -> idq/1
  Fdq/1 -> Demux1/1
  Interpolation Using Prelookup/1 -> Product6/2

== system Motor_ctrl_INST/Power block - Inverter + Motor/Circuital/Motor model/CCG model/Motor Model/Inverse Flux Maps/3D LUTs/Variant Subsystem/PM-SyR ==
  Fdq : Inport
  theta_elt : Inport  Port=2
  Abs3 : Abs  SaturateOnIntegerOverflow=off
  Demux1 : Demux  Outputs=2
  Interpolation Using Prelookup : Interpolation_n-D  NumberOfTableDimensions=3  Table=T_dqt  LookupTableObject=T_th  RequireIndexFractionAsBus=on  InternalRulePriority=Speed
      settings: InputPortMap=u0,u1,u2
  Interpolation Using Prelookup3 : Interpolation_n-D  NumberOfTableDimensions=3  Table=Id_dqt  RequireIndexFractionAsBus=on  InternalRulePriority=Speed
      settings: InputPortMap=u0,u1,u2
  Interpolation Using Prelookup4 : Interpolation_n-D  NumberOfTableDimensions=3  Table=Iq_dqt  RequireIndexFractionAsBus=on  InternalRulePriority=Speed
      settings: InputPortMap=u0,u1,u2
  MATLAB Function2 : MATLAB Function  TreatAsAtomicUnit=on
  Mux1 : Mux  Inputs=2
  Prelookup1 : PreLookup  BreakpointsData=Fd_v  OutputSelection=Index and fraction as bus  ExtrapMethod=Linear
  Prelookup2 : PreLookup  BreakpointsData=Fq_v  OutputSelection=Index and fraction as bus  ExtrapMethod=Linear
  Prelookup6 : PreLookup  BreakpointsData=th_v  OutputSelection=Index and fraction as bus  ExtrapMethod=Linear
  Product : Product
  Product6 : Product
  Sign2 : Signum
  th_lim : Saturate  UpperLimit=th_max  LowerLimit=th_min  ZeroCross=off
  idq : Outport
  T : Outport  Port=2
  wires:
  Sign2/1 -> Product6/1, Product/1
  Interpolation Using Prelookup3/1 -> Product/2
  ? -> ?
  theta_elt/1 -> MATLAB Function2/1(th_rad)
  Product/1 -> Mux1/1
  Interpolation Using Prelookup4/1 -> Mux1/2
  Product6/1 -> T/1
  Abs3/1 -> Prelookup1/1  "fd"
  MATLAB Function2/1(th_deg) -> th_lim/1
  [bus_d] -> Interpolation Using Prelookup3/2
  [bus_d] -> Interpolation Using Prelookup4/2
  Prelookup1/1 -> [bus_d]
  [bus_q] -> Interpolation Using Prelookup/1
  Demux1/2 -> Prelookup2/1  "fq"
  [bus_th] -> Interpolation Using Prelookup/3
  [bus_q] -> Interpolation Using Prelookup4/1
  [bus_d] -> Interpolation Using Prelookup/2
  [bus_q] -> Interpolation Using Prelookup3/1
  [bus_th] -> Interpolation Using Prelookup4/3
  Demux1/1 -> Sign2/1, Abs3/1  "fd"
  th_lim/1 -> Prelookup6/1
  Prelookup6/1 -> [bus_th]
  [bus_th] -> Interpolation Using Prelookup3/3
  Prelookup2/1 -> [bus_q]
  Mux1/1 -> idq/1
  Fdq/1 -> Demux1/1
  Interpolation Using Prelookup/1 -> Product6/2

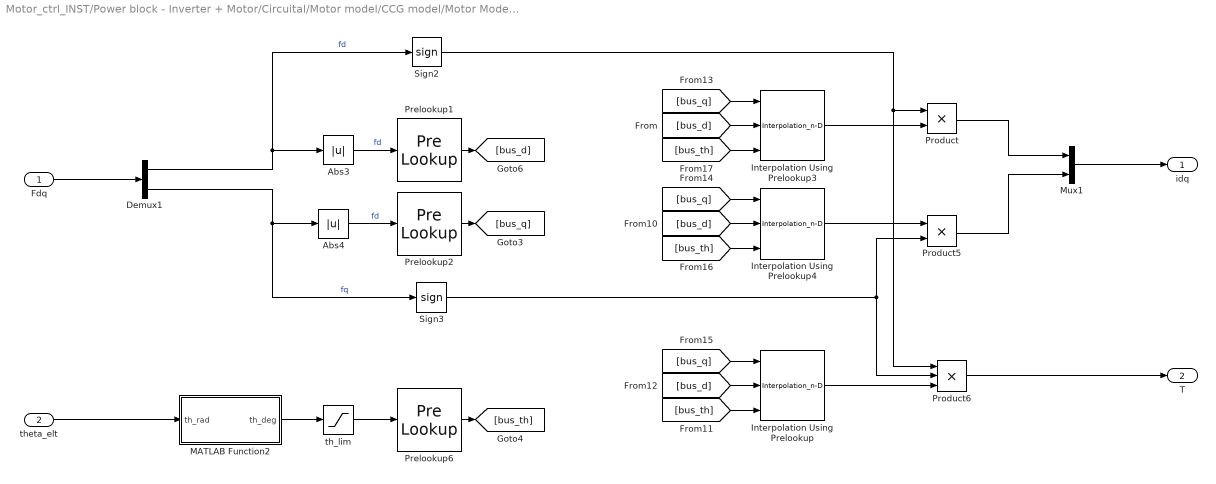
== system Motor_ctrl_INST/Power block - Inverter + Motor/Circuital/Motor model/CCG model/Motor Model/Inverse Flux Maps/3D LUTs/Variant Subsystem/SyR ==
  Fdq : Inport
  theta_elt : Inport  Port=2
  Abs3 : Abs  SaturateOnIntegerOverflow=off
  Abs4 : Abs  SaturateOnIntegerOverflow=off
  Demux1 : Demux  Outputs=2
  Interpolation Using Prelookup : Interpolation_n-D  NumberOfTableDimensions=3  Table=T_dqt  LookupTableObject=T_th  RequireIndexFractionAsBus=on  InternalRulePriority=Speed
      settings: InputPortMap=u0,u1,u2
  Interpolation Using Prelookup3 : Interpolation_n-D  NumberOfTableDimensions=3  Table=Id_dqt  RequireIndexFractionAsBus=on  InternalRulePriority=Speed
      settings: InputPortMap=u0,u1,u2
  Interpolation Using Prelookup4 : Interpolation_n-D  NumberOfTableDimensions=3  Table=Iq_dqt  RequireIndexFractionAsBus=on  InternalRulePriority=Speed
      settings: InputPortMap=u0,u1,u2
  MATLAB Function2 : MATLAB Function  TreatAsAtomicUnit=on
  Mux1 : Mux  Inputs=2
  Prelookup1 : PreLookup  BreakpointsData=Fd_v  OutputSelection=Index and fraction as bus  ExtrapMethod=Linear
  Prelookup2 : PreLookup  BreakpointsData=Fq_v  OutputSelection=Index and fraction as bus  ExtrapMethod=Linear
  Prelookup6 : PreLookup  BreakpointsData=th_v  OutputSelection=Index and fraction as bus  ExtrapMethod=Linear
  Product : Product
  Product5 : Product
  Product6 : Product  Inputs=3
  Sign2 : Signum
  Sign3 : Signum
  th_lim : Saturate  UpperLimit=th_max  LowerLimit=th_min  ZeroCross=off
  idq : Outport
  T : Outport  Port=2
  wires:
  th_lim/1 -> Prelookup6/1
  [bus_q] -> Interpolation Using Prelookup3/1
  Demux1/1 -> Sign2/1, Abs3/1  "fd"
  Prelookup6/1 -> [bus_th]
  Prelookup2/1 -> [bus_q]
  [bus_th] -> Interpolation Using Prelookup4/3
  [bus_q] -> Interpolation Using Prelookup4/1
  Fdq/1 -> Demux1/1
  [bus_q] -> Interpolation Using Prelookup/1
  [bus_th] -> Interpolation Using Prelookup/3
  [bus_d] -> Interpolation Using Prelookup4/2
  [bus_d] -> Interpolation Using Prelookup/2
  Demux1/2 -> Sign3/1, Abs4/1  "fq"
  Prelookup1/1 -> [bus_d]
  theta_elt/1 -> MATLAB Function2/1(th_rad)
  [bus_th] -> Interpolation Using Prelookup3/3
  [bus_d] -> Interpolation Using Prelookup3/2
  MATLAB Function2/1(th_deg) -> th_lim/1
  Abs3/1 -> Prelookup1/1  "fd"
  Abs4/1 -> Prelookup2/1  "fd"
  Interpolation Using Prelookup3/1 -> Product/2
  Sign2/1 -> Product6/1, Product/1
  Interpolation Using Prelookup4/1 -> Product5/1
  Sign3/1 -> Product6/2, Product5/2
  Product/1 -> Mux1/1
  Product5/1 -> Mux1/2
  Mux1/1 -> idq/1
  Interpolation Using Prelookup/1 -> Product6/3
  Product6/1 -> T/1

== system Motor_ctrl_INST/Power block - Inverter + Motor/Circuital/Motor model/CCG model/Motor Model/Iron Losses Maps/Iron Losses/Iron loss Maps/Speed Adaptation ==
  n_m : Inport
  Constant : Constant  Value=n0
  Constant1 : Constant  Value=expC
  Constant2 : Constant  Value=expH
  Constant3 : Constant  Value=expPM
  Divide : Product  Inputs=*/
  Math Function : Math  Operator=pow  SignedPower=on
  Math Function1 : Math  Operator=pow  SignedPower=on
  Math Function2 : Math  Operator=pow  SignedPower=on
  H : Outport
  C : Outport  Port=2
  PM : Outport  Port=3
  wires:
  Math Function2/1 -> PM/1
  Math Function/1 -> H/1
  Constant1/1 -> Math Function1/2
  Divide/1 -> Math Function/1, Math Function1/1, Math Function2/1
  Math Function1/1 -> C/1
  Constant/1 -> Divide/2
  Constant2/1 -> Math Function/2
  Constant3/1 -> Math Function2/2
  n_m/1 -> Divide/1

== system Motor_ctrl_INST/Power block - Inverter + Motor/Noncircuital/FM/Motor Model/Inverse Flux Maps/2D LUT/dq Model/IPM/Fdq -> idq ==
  Fdq : Inport
  1-D Lookup Table : Lookup_n-D  NumberOfTableDimensions=1  BreakpointsForDimension1=fD_vct_ref  Table=fQ_vct_max  InternalRulePriority=Speed  RndMeth=Simplest
  Abs1 : Abs  SaturateOnIntegerOverflow=off
  Bias : Bias  Bias=-fD_vct_ref(1)  SaturateOnIntegerOverflow=off
  Constant : Constant  Value=fD_vct_ref(end)-fD_vct_ref(1)
  Demux : Demux  Outputs=2
  Divide : Product  Inputs=*/
  Divide1 : Product  Inputs=/*
  Id_pu : Lookup_n-D  BreakpointsForDimension1=fQ_pu_norm(:,1)  BreakpointsForDimension2=fD_pu_norm(1,:)  Table=iD_pu_norm  InternalRulePriority=Speed  RndMeth=Simplest
      settings: InputPortMap=u0,u1
  Iq_pu : Lookup_n-D  BreakpointsForDimension1=fQ_pu_norm(:,1)  BreakpointsForDimension2=fD_pu_norm(1,:)  Table=iQ_pu_norm  InternalRulePriority=Speed  RndMeth=Simplest
      settings: InputPortMap=u0,u1
  Mux : Mux  Inputs=2
  Product1 : Product
  Saturation : Saturate  UpperLimit=fD_vct_ref(end)  LowerLimit=fD_vct_ref(1)
  Saturation Dynamic : simulink/Discontinuities/Saturation Dynamic  OutMin=[]  OutMax=[]  OutDataTypeStr=Inherit: Same as second input  OutDataType=fixdt(1, 16)  OutScaling=2^-10  DoSatur=off
  Sign1 : Signum
  Torque calculation : Subsystem
  idq : Outport
  T : Outport  Port=2
  wires:
  Mux/1 -> Torque calculation/1(Idq), idq/1
  Iq_pu/1 -> Product1/1
  Torque calculation/1(Tm) -> T/1
  Sign1/1 -> Product1/2
  1-D Lookup Table/1 -> Divide1/1, Saturation Dynamic/1
  Divide/1 -> Iq_pu/2, Id_pu/2
  Saturation Dynamic/1 -> Divide1/2
  Abs1/1 -> Saturation Dynamic/3, Saturation Dynamic/2
  Divide1/1 -> Id_pu/1, Iq_pu/1
  Demux/1 -> Saturation/1
  Constant/1 -> Divide/2
  Product1/1 -> Mux/2  "iq_pu"
  Demux/2 -> Sign1/1, Abs1/1
  Fdq/1 -> Torque calculation/2(Fdq), Demux/1
  Id_pu/1 -> Mux/1  "iq_pu"
  Saturation/1 -> Bias/1, 1-D Lookup Table/1
  Bias/1 -> Divide/1

== system Motor_ctrl_INST/Power block - Inverter + Motor/Noncircuital/FM/Motor Model/Inverse Flux Maps/2D LUT/dq Model/IPM/Subsystem1 ==
  theta_r : Inport
  Gain1 : Gain  Gain=p
  Mux3 : Mux  Inputs=2
  Scope : Scope
  Scope1 : Scope
  Sin : Trigonometry
  Sin1 : Trigonometry  Operator=cos
  SinCos : Outport
  wires:
  Sin1/1 -> Mux3/2
  Sin/1 -> Mux3/1
  Mux3/1 -> Scope/1, SinCos/1
  Gain1/1 -> Scope1/1, Sin/1, Sin1/1
  theta_r/1 -> Gain1/1

== system Motor_ctrl_INST/Power block - Inverter + Motor/Noncircuital/FM/Motor Model/Inverse Flux Maps/2D LUT/dq Model/IPM/ab->dq1 ==
  X_ab : Inport
  sin,cos : Inport  Port=2
  Demux : Demux  Outputs=2
  Demux1 : Demux  Outputs=2
  Mux : Mux  Commented=on  Inputs=2
  Mux1 : Mux  Commented=on  Inputs=2
  Mux2 : Mux  Inputs=2
  Product{,1..3} (4 alike) : Product
  Subtract : Sum
  Subtract1 : Sum  Inputs=-+
  X_d : Fcn  Commented=on  Expr=u(1)*u(4) + u(2)*u(3)
  X_q : Fcn  Commented=on  Expr=- u(1)*u(3) + u(2)*u(4)
  X_dq : Outport  InitialOutput=0
  wires:
  X_q/1 -> Mux1/2
  X_d/1 -> Mux1/1
  Mux/1 -> X_q/1, X_d/1
  Demux1/2 -> Product1/2, Product/2
  Demux/2 -> Product1/1, Product2/1
  Demux1/1 -> Product3/2, Product2/2
  Product/1 -> Subtract/1
  Product2/1 -> Subtract/2
  Demux/1 -> Product3/1, Product/1
  Product3/1 -> Subtract1/1
  Product1/1 -> Subtract1/2
  Subtract/1 -> Mux2/1
  Subtract1/1 -> Mux2/2
  X_ab/1 -> Demux/1
  sin,cos/1 -> Demux1/1
  Mux2/1 -> X_dq/1

== system Motor_ctrl_INST/Power block - Inverter + Motor/Noncircuital/FM/Motor Model/Inverse Flux Maps/2D LUT/dq Model/IPM/abc->ab0 ==
  eabc : Inport
  Demux1 : Demux  Outputs=3
  Gain : Gain  Gain=0.5
  Gain1 : Gain  Gain=2/3
  Gain2 : Gain  Gain=1/sqrt(3)
  Gain3 : Gain  Gain=1/3
  Mux1 : Mux  Inputs=3
  Subtract : Sum  Inputs=+-
  Subtract1 : Sum
  Subtract2 : Sum  Inputs=+-
  Subtract3 : Sum  Inputs=+++
  eab0 : Outport
  wires:
  Subtract1/1 -> Gain/1
  Subtract/1 -> Gain1/1
  Demux1/2 -> Subtract3/2, Subtract2/1, Subtract1/1
  Subtract2/1 -> Gain2/1
  Subtract3/1 -> Gain3/1
  Gain1/1 -> Mux1/1
  Demux1/1 -> Subtract/1, Subtract3/1
  Gain3/1 -> Mux1/3
  Gain2/1 -> Mux1/2
  Gain/1 -> Subtract/2
  Mux1/1 -> eab0/1
  Demux1/3 -> Subtract3/3, Subtract2/2, Subtract1/2
  eabc/1 -> Demux1/1

== system Motor_ctrl_INST/Power block - Inverter + Motor/Noncircuital/FM/Motor Model/Inverse Flux Maps/2D LUT/dq Model/PM-SyR/Fdq -> idq ==
  Fdq : Inport
  1-D Lookup Table : Lookup_n-D  NumberOfTableDimensions=1  BreakpointsForDimension1=fQ_vct_ref  Table=fD_vct_max  InternalRulePriority=Speed  RndMeth=Simplest
  Abs : Abs  SaturateOnIntegerOverflow=off
  Bias : Bias  Bias=-fQ_vct_ref(1)  SaturateOnIntegerOverflow=off
  Constant : Constant  Value=fQ_vct_ref(end)-fQ_vct_ref(1)
  Demux : Demux  Outputs=2
  Divide : Product  Inputs=*/
  Divide1 : Product  Inputs=/*
  Id_pu : Lookup_n-D  BreakpointsForDimension1=fQ_pu_norm(:,1)  BreakpointsForDimension2=fD_pu_norm(1,:)  Table=iD_pu_norm  InternalRulePriority=Speed  RndMeth=Simplest
      settings: InputPortMap=u0,u1
  Iq_pu : Lookup_n-D  BreakpointsForDimension1=fQ_pu_norm(:,1)  BreakpointsForDimension2=fD_pu_norm(1,:)  Table=iQ_pu_norm  InternalRulePriority=Speed  RndMeth=Simplest
      settings: InputPortMap=u0,u1
  Mux : Mux  Inputs=2
  Product2 : Product
  Saturation : Saturate  UpperLimit=fQ_vct_ref(end)  LowerLimit=fQ_vct_ref(1)
  Saturation Dynamic : simulink/Discontinuities/Saturation Dynamic  OutMin=[]  OutMax=[]  OutDataTypeStr=Inherit: Same as second input  OutDataType=fixdt(1, 16)  OutScaling=2^-10  DoSatur=off
  Sign2 : Signum
  Torque calculation : Subsystem
  idq : Outport
  T : Outport  Port=2
  wires:
  Sign2/1 -> Product2/1
  Constant/1 -> Divide/2
  Abs/1 -> Saturation Dynamic/3, Saturation Dynamic/2
  Iq_pu/1 -> Mux/2  "iq_pu"
  Torque calculation/1(Tm) -> T/1
  Divide/1 -> Iq_pu/1, Id_pu/1
  Bias/1 -> Divide/1
  1-D Lookup Table/1 -> Divide1/1, Saturation Dynamic/1
  Saturation/1 -> Bias/1, 1-D Lookup Table/1
  Mux/1 -> idq/1, Torque calculation/1(Idq)
  Id_pu/1 -> Product2/2
  Demux/1 -> Sign2/1, Abs/1
  Divide1/1 -> Id_pu/2, Iq_pu/2
  Demux/2 -> Saturation/1
  Fdq/1 -> Torque calculation/2(Fdq), Demux/1
  Product2/1 -> Mux/1  "id_pu"
  Saturation Dynamic/1 -> Divide1/2

== system Motor_ctrl_INST/Power block - Inverter + Motor/Noncircuital/FM/Motor Model/Inverse Flux Maps/2D LUT/dq Model/PM-SyR/Subsystem1 ==
  theta_r : Inport
  Gain1 : Gain  Gain=p
  Mux3 : Mux  Inputs=2
  Scope : Scope
  Scope1 : Scope
  Sin : Trigonometry
  Sin1 : Trigonometry  Operator=cos
  SinCos : Outport
  wires:
  Sin1/1 -> Mux3/2
  Sin/1 -> Mux3/1
  Mux3/1 -> Scope/1, SinCos/1
  Gain1/1 -> Scope1/1, Sin/1, Sin1/1
  theta_r/1 -> Gain1/1

== system Motor_ctrl_INST/Power block - Inverter + Motor/Noncircuital/FM/Motor Model/Inverse Flux Maps/2D LUT/dq Model/PM-SyR/ab->dq1 ==
  X_ab : Inport
  sin,cos : Inport  Port=2
  Demux : Demux  Outputs=2
  Demux1 : Demux  Outputs=2
  Mux : Mux  Commented=on  Inputs=2
  Mux1 : Mux  Commented=on  Inputs=2
  Mux2 : Mux  Inputs=2
  Product{,1..3} (4 alike) : Product
  Subtract : Sum
  Subtract1 : Sum  Inputs=-+
  X_d : Fcn  Commented=on  Expr=u(1)*u(4) + u(2)*u(3)
  X_q : Fcn  Commented=on  Expr=- u(1)*u(3) + u(2)*u(4)
  X_dq : Outport  InitialOutput=0
  wires:
  X_q/1 -> Mux1/2
  X_d/1 -> Mux1/1
  Mux/1 -> X_q/1, X_d/1
  Demux1/2 -> Product1/2, Product/2
  Demux/2 -> Product1/1, Product2/1
  Demux1/1 -> Product3/2, Product2/2
  Product/1 -> Subtract/1
  Product2/1 -> Subtract/2
  Demux/1 -> Product3/1, Product/1
  Product3/1 -> Subtract1/1
  Product1/1 -> Subtract1/2
  Subtract/1 -> Mux2/1
  Subtract1/1 -> Mux2/2
  X_ab/1 -> Demux/1
  sin,cos/1 -> Demux1/1
  Mux2/1 -> X_dq/1

== system Motor_ctrl_INST/Power block - Inverter + Motor/Noncircuital/FM/Motor Model/Inverse Flux Maps/2D LUT/dq Model/PM-SyR/abc->ab0 ==
  eabc : Inport
  Demux1 : Demux  Outputs=3
  Gain : Gain  Gain=0.5
  Gain1 : Gain  Gain=2/3
  Gain2 : Gain  Gain=1/sqrt(3)
  Gain3 : Gain  Gain=1/3
  Mux1 : Mux  Inputs=3
  Subtract : Sum  Inputs=+-
  Subtract1 : Sum
  Subtract2 : Sum  Inputs=+-
  Subtract3 : Sum  Inputs=+++
  eab0 : Outport
  wires:
  Subtract1/1 -> Gain/1
  Subtract/1 -> Gain1/1
  Demux1/2 -> Subtract3/2, Subtract2/1, Subtract1/1
  Subtract2/1 -> Gain2/1
  Subtract3/1 -> Gain3/1
  Gain1/1 -> Mux1/1
  Demux1/1 -> Subtract/1, Subtract3/1
  Gain3/1 -> Mux1/3
  Gain2/1 -> Mux1/2
  Gain/1 -> Subtract/2
  Mux1/1 -> eab0/1
  Demux1/3 -> Subtract3/3, Subtract2/2, Subtract1/2
  eabc/1 -> Demux1/1
